simulink model "ULInjurySubject_Biphasic_1Hz_08102023"  (R2023a)
settings: Solver=VariableStepAuto  StartTime=0.0  StopTime=2000  RelTol=1e-3
values from neighbouring files (symbols this model uses):
  Cn = 1    [Inhibitory_excitatory_ULInjury_1Hz_08102023.m]    (also in Inhibitory_excitatory_ULInjury_30Hz_08102023.m; InitialExcitatoryInhibitoryNeurons_Healthy08062023.m; InitialExcitatoryInhibitoryULInjured_08102023_DSD.m)
  EKEx = -90    [Inhibitory_excitatory_ULInjury_1Hz_08102023.m]    (also in Inhibitory_excitatory_ULInjury_30Hz_08102023.m; InitialExcitatoryInhibitoryNeurons_Healthy08062023.m; InitialExcitatoryInhibitoryULInjured_08102023_DSD.m)
  EKIn = -90    [Inhibitory_excitatory_ULInjury_1Hz_08102023.m]    (also in Inhibitory_excitatory_ULInjury_30Hz_08102023.m; InitialExcitatoryInhibitoryNeurons_Healthy08062023.m; InitialExcitatoryInhibitoryULInjured_08102023_DSD.m)
  ELEx = -65    [Inhibitory_excitatory_ULInjury_1Hz_08102023.m]    (also in Inhibitory_excitatory_ULInjury_30Hz_08102023.m; InitialExcitatoryInhibitoryNeurons_Healthy08062023.m; InitialExcitatoryInhibitoryULInjured_08102023_DSD.m)
  ELIn = -65    [Inhibitory_excitatory_ULInjury_1Hz_08102023.m]    (also in Inhibitory_excitatory_ULInjury_30Hz_08102023.m; InitialExcitatoryInhibitoryNeurons_Healthy08062023.m; InitialExcitatoryInhibitoryULInjured_08102023_DSD.m)
  ENaEx = 60    [Inhibitory_excitatory_ULInjury_1Hz_08102023.m]    (also in Inhibitory_excitatory_ULInjury_30Hz_08102023.m; InitialExcitatoryInhibitoryNeurons_Healthy08062023.m; InitialExcitatoryInhibitoryULInjured_08102023_DSD.m)
  ENaIn = 55    [Inhibitory_excitatory_ULInjury_1Hz_08102023.m]    (also in Inhibitory_excitatory_ULInjury_30Hz_08102023.m; InitialExcitatoryInhibitoryNeurons_Healthy08062023.m; InitialExcitatoryInhibitoryULInjured_08102023_DSD.m)
  ErestE = -65    [Inhibitory_excitatory_ULInjury_1Hz_08102023.m]    (also in Inhibitory_excitatory_ULInjury_30Hz_08102023.m; InitialExcitatoryInhibitoryNeurons_Healthy08062023.m; InitialExcitatoryInhibitoryULInjured_08102023_DSD.m)
  ErestIn = -64    [Inhibitory_excitatory_ULInjury_1Hz_08102023.m]    (also in Inhibitory_excitatory_ULInjury_30Hz_08102023.m; InitialExcitatoryInhibitoryNeurons_Healthy08062023.m; InitialExcitatoryInhibitoryULInjured_08102023_DSD.m)
  ESynE = -10    [Inhibitory_excitatory_ULInjury_1Hz_08102023.m]    (also in Inhibitory_excitatory_ULInjury_30Hz_08102023.m; InitialExcitatoryInhibitoryNeurons_Healthy08062023.m; InitialExcitatoryInhibitoryULInjured_08102023_DSD.m)
  ESynE2 = -10    [Inhibitory_excitatory_ULInjury_1Hz_08102023.m]    (also in Inhibitory_excitatory_ULInjury_30Hz_08102023.m; InitialExcitatoryInhibitoryNeurons_Healthy08062023.m; InitialExcitatoryInhibitoryULInjured_08102023_DSD.m)
  ESynE3 = -10    [Inhibitory_excitatory_ULInjury_1Hz_08102023.m]    (also in Inhibitory_excitatory_ULInjury_30Hz_08102023.m; InitialExcitatoryInhibitoryNeurons_Healthy08062023.m; InitialExcitatoryInhibitoryULInjured_08102023_DSD.m)
  ESynE4 = -10    [Inhibitory_excitatory_ULInjury_1Hz_08102023.m]    (also in Inhibitory_excitatory_ULInjury_30Hz_08102023.m; InitialExcitatoryInhibitoryNeurons_Healthy08062023.m; InitialExcitatoryInhibitoryULInjured_08102023_DSD.m)
  ESynE5 = -10    [Inhibitory_excitatory_ULInjury_1Hz_08102023.m]    (also in Inhibitory_excitatory_ULInjury_30Hz_08102023.m; InitialExcitatoryInhibitoryNeurons_Healthy08062023.m; InitialExcitatoryInhibitoryULInjured_08102023_DSD.m)
  ESynE610 = -24    [Inhibitory_excitatory_ULInjury_1Hz_08102023.m]    (also in Inhibitory_excitatory_ULInjury_30Hz_08102023.m; InitialExcitatoryInhibitoryNeurons_Healthy08062023.m; InitialExcitatoryInhibitoryULInjured_08102023_DSD.m)
  ESynE6p = -10    [Inhibitory_excitatory_ULInjury_1Hz_08102023.m]    (also in Inhibitory_excitatory_ULInjury_30Hz_08102023.m; InitialExcitatoryInhibitoryNeurons_Healthy08062023.m; InitialExcitatoryInhibitoryULInjured_08102023_DSD.m)
  ESynI2 = -80    [Inhibitory_excitatory_ULInjury_1Hz_08102023.m]    (also in Inhibitory_excitatory_ULInjury_30Hz_08102023.m; InitialExcitatoryInhibitoryNeurons_Healthy08062023.m; InitialExcitatoryInhibitoryULInjured_08102023_DSD.m)
  ESynI3 = -80    [Inhibitory_excitatory_ULInjury_1Hz_08102023.m]    (also in Inhibitory_excitatory_ULInjury_30Hz_08102023.m; InitialExcitatoryInhibitoryNeurons_Healthy08062023.m; InitialExcitatoryInhibitoryULInjured_08102023_DSD.m)
  ESynI5 = -80    [Inhibitory_excitatory_ULInjury_1Hz_08102023.m]    (also in Inhibitory_excitatory_ULInjury_30Hz_08102023.m; InitialExcitatoryInhibitoryNeurons_Healthy08062023.m; InitialExcitatoryInhibitoryULInjured_08102023_DSD.m)
  ESynI6p = -82    [Inhibitory_excitatory_ULInjury_1Hz_08102023.m]    (also in Inhibitory_excitatory_ULInjury_30Hz_08102023.m; InitialExcitatoryInhibitoryNeurons_Healthy08062023.m; InitialExcitatoryInhibitoryULInjured_08102023_DSD.m)
  Exh0 = ahEx(V0)./(ahEx(V0)+bhEx(V0))    [Inhibitory_excitatory_ULInjury_1Hz_08102023.m]    (also in Inhibitory_excitatory_ULInjury_30Hz_08102023.m; InitialExcitatoryInhibitoryNeurons_Healthy08062023.m; InitialExcitatoryInhibitoryULInjured_08102023_DSD.m)
  Exm0 = amEx(V0)./(amEx(V0)+bmEx(V0))    [Inhibitory_excitatory_ULInjury_1Hz_08102023.m]    (also in Inhibitory_excitatory_ULInjury_30Hz_08102023.m; InitialExcitatoryInhibitoryNeurons_Healthy08062023.m; InitialExcitatoryInhibitoryULInjured_08102023_DSD.m)
  Exn0 = anEx(V0)./(anEx(V0)+bnEx(V0))    [Inhibitory_excitatory_ULInjury_1Hz_08102023.m]    (also in Inhibitory_excitatory_ULInjury_30Hz_08102023.m; InitialExcitatoryInhibitoryNeurons_Healthy08062023.m; InitialExcitatoryInhibitoryULInjured_08102023_DSD.m)
  gKEx = 100    [Inhibitory_excitatory_ULInjury_1Hz_08102023.m]    (also in Inhibitory_excitatory_ULInjury_30Hz_08102023.m; InitialExcitatoryInhibitoryNeurons_Healthy08062023.m; InitialExcitatoryInhibitoryULInjured_08102023_DSD.m)
  gKIn = 9    [Inhibitory_excitatory_ULInjury_1Hz_08102023.m]    (also in Inhibitory_excitatory_ULInjury_30Hz_08102023.m; InitialExcitatoryInhibitoryNeurons_Healthy08062023.m; InitialExcitatoryInhibitoryULInjured_08102023_DSD.m)
  gLEx = 0.1    [Inhibitory_excitatory_ULInjury_1Hz_08102023.m]    (also in Inhibitory_excitatory_ULInjury_30Hz_08102023.m; InitialExcitatoryInhibitoryNeurons_Healthy08062023.m; InitialExcitatoryInhibitoryULInjured_08102023_DSD.m)
  gLIn = 0.1    [Inhibitory_excitatory_ULInjury_1Hz_08102023.m]    (also in Inhibitory_excitatory_ULInjury_30Hz_08102023.m; InitialExcitatoryInhibitoryNeurons_Healthy08062023.m; InitialExcitatoryInhibitoryULInjured_08102023_DSD.m)
  gNaEx = 30    [Inhibitory_excitatory_ULInjury_1Hz_08102023.m]    (also in Inhibitory_excitatory_ULInjury_30Hz_08102023.m; InitialExcitatoryInhibitoryNeurons_Healthy08062023.m; InitialExcitatoryInhibitoryULInjured_08102023_DSD.m)
  gNaIn = 35    [Inhibitory_excitatory_ULInjury_1Hz_08102023.m]    (also in Inhibitory_excitatory_ULInjury_30Hz_08102023.m; InitialExcitatoryInhibitoryNeurons_Healthy08062023.m; InitialExcitatoryInhibitoryULInjured_08102023_DSD.m)
  gSynE = 0.08    [Inhibitory_excitatory_ULInjury_1Hz_08102023.m]    (also in Inhibitory_excitatory_ULInjury_30Hz_08102023.m; InitialExcitatoryInhibitoryNeurons_Healthy08062023.m; InitialExcitatoryInhibitoryULInjured_08102023_DSD.m)
  gSynE2 = 0.08    [Inhibitory_excitatory_ULInjury_1Hz_08102023.m]    (also in Inhibitory_excitatory_ULInjury_30Hz_08102023.m; InitialExcitatoryInhibitoryNeurons_Healthy08062023.m; InitialExcitatoryInhibitoryULInjured_08102023_DSD.m)
  gSynE3 = 0.08    [Inhibitory_excitatory_ULInjury_1Hz_08102023.m]    (also in Inhibitory_excitatory_ULInjury_30Hz_08102023.m; InitialExcitatoryInhibitoryNeurons_Healthy08062023.m; InitialExcitatoryInhibitoryULInjured_08102023_DSD.m)
  gSynE4 = 0.08    [Inhibitory_excitatory_ULInjury_1Hz_08102023.m]    (also in Inhibitory_excitatory_ULInjury_30Hz_08102023.m; InitialExcitatoryInhibitoryNeurons_Healthy08062023.m; InitialExcitatoryInhibitoryULInjured_08102023_DSD.m)
  gSynE5 = 0.08    [Inhibitory_excitatory_ULInjury_1Hz_08102023.m]    (also in Inhibitory_excitatory_ULInjury_30Hz_08102023.m; InitialExcitatoryInhibitoryNeurons_Healthy08062023.m; InitialExcitatoryInhibitoryULInjured_08102023_DSD.m)
  gSynE6 = 0.08    [Inhibitory_excitatory_ULInjury_1Hz_08102023.m]    (also in Inhibitory_excitatory_ULInjury_30Hz_08102023.m; InitialExcitatoryInhibitoryNeurons_Healthy08062023.m; InitialExcitatoryInhibitoryULInjured_08102023_DSD.m)
  gSynI2 = 0.12    [Inhibitory_excitatory_ULInjury_1Hz_08102023.m]    (also in Inhibitory_excitatory_ULInjury_30Hz_08102023.m; InitialExcitatoryInhibitoryNeurons_Healthy08062023.m; InitialExcitatoryInhibitoryULInjured_08102023_DSD.m)
  gSynI3 = 0.12    [Inhibitory_excitatory_ULInjury_1Hz_08102023.m]    (also in Inhibitory_excitatory_ULInjury_30Hz_08102023.m; InitialExcitatoryInhibitoryNeurons_Healthy08062023.m; InitialExcitatoryInhibitoryULInjured_08102023_DSD.m)
  gSynI5 = 0.12    [Inhibitory_excitatory_ULInjury_1Hz_08102023.m]    (also in Inhibitory_excitatory_ULInjury_30Hz_08102023.m; InitialExcitatoryInhibitoryNeurons_Healthy08062023.m; InitialExcitatoryInhibitoryULInjured_08102023_DSD.m)
  gSynI6 = 0.12    [Inhibitory_excitatory_ULInjury_1Hz_08102023.m]    (also in Inhibitory_excitatory_ULInjury_30Hz_08102023.m; InitialExcitatoryInhibitoryNeurons_Healthy08062023.m; InitialExcitatoryInhibitoryULInjured_08102023_DSD.m)
  Inh0 = ahIn(ErestIn)./(ahIn(ErestIn)+bhIn(ErestIn))    [Inhibitory_excitatory_ULInjury_1Hz_08102023.m]    (also in Inhibitory_excitatory_ULInjury_30Hz_08102023.m; InitialExcitatoryInhibitoryNeurons_Healthy08062023.m; InitialExcitatoryInhibitoryULInjured_08102023_DSD.m)
  Inm0 = amIn(ErestIn)./(amIn(ErestIn)+bmIn(ErestIn))    [Inhibitory_excitatory_ULInjury_1Hz_08102023.m]    (also in Inhibitory_excitatory_ULInjury_30Hz_08102023.m; InitialExcitatoryInhibitoryNeurons_Healthy08062023.m; InitialExcitatoryInhibitoryULInjured_08102023_DSD.m)
  Inn0 = anIn(ErestIn)./(anIn(ErestIn)+bnIn(ErestIn))    [Inhibitory_excitatory_ULInjury_1Hz_08102023.m]    (also in Inhibitory_excitatory_ULInjury_30Hz_08102023.m; InitialExcitatoryInhibitoryNeurons_Healthy08062023.m; InitialExcitatoryInhibitoryULInjured_08102023_DSD.m)
  TawIExt = 30    [Inhibitory_excitatory_ULInjury_1Hz_08102023.m]    (also in Inhibitory_excitatory_ULInjury_30Hz_08102023.m; InitialExcitatoryInhibitoryNeurons_Healthy08062023.m = 200; InitialExcitatoryInhibitoryULInjured_08102023_DSD.m = 200)
  TawIExtE = 30    [Inhibitory_excitatory_ULInjury_1Hz_08102023.m]    (also in Inhibitory_excitatory_ULInjury_30Hz_08102023.m; InitialExcitatoryInhibitoryNeurons_Healthy08062023.m = 1; InitialExcitatoryInhibitoryULInjured_08102023_DSD.m = 10)
  TawSynE = 5    [Inhibitory_excitatory_ULInjury_1Hz_08102023.m]    (also in Inhibitory_excitatory_ULInjury_30Hz_08102023.m; InitialExcitatoryInhibitoryNeurons_Healthy08062023.m; InitialExcitatoryInhibitoryULInjured_08102023_DSD.m)
  TawSynE10 = 5    [Inhibitory_excitatory_ULInjury_1Hz_08102023.m]    (also in Inhibitory_excitatory_ULInjury_30Hz_08102023.m; InitialExcitatoryInhibitoryNeurons_Healthy08062023.m; InitialExcitatoryInhibitoryULInjured_08102023_DSD.m = 3)
  TawSynE2 = 11    [Inhibitory_excitatory_ULInjury_1Hz_08102023.m]    (also in Inhibitory_excitatory_ULInjury_30Hz_08102023.m; InitialExcitatoryInhibitoryNeurons_Healthy08062023.m = 12; InitialExcitatoryInhibitoryULInjured_08102023_DSD.m = 5)
  TawSynE3 = 10    [Inhibitory_excitatory_ULInjury_1Hz_08102023.m]    (also in Inhibitory_excitatory_ULInjury_30Hz_08102023.m; InitialExcitatoryInhibitoryNeurons_Healthy08062023.m = 18; InitialExcitatoryInhibitoryULInjured_08102023_DSD.m = 8)
  TawSynE4 = 6    [Inhibitory_excitatory_ULInjury_1Hz_08102023.m]    (also in Inhibitory_excitatory_ULInjury_30Hz_08102023.m; InitialExcitatoryInhibitoryNeurons_Healthy08062023.m; InitialExcitatoryInhibitoryULInjured_08102023_DSD.m)
  TawSynE41 = 14    [Inhibitory_excitatory_ULInjury_1Hz_08102023.m]    (also in Inhibitory_excitatory_ULInjury_30Hz_08102023.m; InitialExcitatoryInhibitoryNeurons_Healthy08062023.m = 15; InitialExcitatoryInhibitoryULInjured_08102023_DSD.m = 6)
  TawSynE5 = 6    [Inhibitory_excitatory_ULInjury_1Hz_08102023.m]    (also in Inhibitory_excitatory_ULInjury_30Hz_08102023.m; InitialExcitatoryInhibitoryNeurons_Healthy08062023.m; InitialExcitatoryInhibitoryULInjured_08102023_DSD.m)
  TawSynE6 = 3    [Inhibitory_excitatory_ULInjury_1Hz_08102023.m]    (also in Inhibitory_excitatory_ULInjury_30Hz_08102023.m; InitialExcitatoryInhibitoryNeurons_Healthy08062023.m; InitialExcitatoryInhibitoryULInjured_08102023_DSD.m)
  TawSynE66E = 5    [Inhibitory_excitatory_ULInjury_1Hz_08102023.m]    (also in Inhibitory_excitatory_ULInjury_30Hz_08102023.m; InitialExcitatoryInhibitoryNeurons_Healthy08062023.m; InitialExcitatoryInhibitoryULInjured_08102023_DSD.m)
  TawSynI2 = 1    [Inhibitory_excitatory_ULInjury_1Hz_08102023.m]    (also in Inhibitory_excitatory_ULInjury_30Hz_08102023.m; InitialExcitatoryInhibitoryNeurons_Healthy08062023.m; InitialExcitatoryInhibitoryULInjured_08102023_DSD.m = 2)
  TawSynI3 = 30    [Inhibitory_excitatory_ULInjury_1Hz_08102023.m]    (also in Inhibitory_excitatory_ULInjury_30Hz_08102023.m; InitialExcitatoryInhibitoryNeurons_Healthy08062023.m = 35; InitialExcitatoryInhibitoryULInjured_08102023_DSD.m)
  TawSynI5 = 4    [Inhibitory_excitatory_ULInjury_1Hz_08102023.m]    (also in Inhibitory_excitatory_ULInjury_30Hz_08102023.m; InitialExcitatoryInhibitoryNeurons_Healthy08062023.m = 1; InitialExcitatoryInhibitoryULInjured_08102023_DSD.m = 1)
  TawSynI6 = 3    [Inhibitory_excitatory_ULInjury_1Hz_08102023.m]    (also in Inhibitory_excitatory_ULInjury_30Hz_08102023.m; InitialExcitatoryInhibitoryNeurons_Healthy08062023.m; InitialExcitatoryInhibitoryULInjured_08102023_DSD.m)
  V0 = -65    [Inhibitory_excitatory_ULInjury_1Hz_08102023.m]    (also in Inhibitory_excitatory_ULInjury_30Hz_08102023.m; InitialExcitatoryInhibitoryNeurons_Healthy08062023.m; InitialExcitatoryInhibitoryULInjured_08102023_DSD.m)
  V0In = -64    [Inhibitory_excitatory_ULInjury_1Hz_08102023.m]    (also in Inhibitory_excitatory_ULInjury_30Hz_08102023.m; InitialExcitatoryInhibitoryNeurons_Healthy08062023.m; InitialExcitatoryInhibitoryULInjured_08102023_DSD.m)
  w10 = 0.035    [Inhibitory_excitatory_ULInjury_1Hz_08102023.m]    (also in Inhibitory_excitatory_ULInjury_30Hz_08102023.m; InitialExcitatoryInhibitoryNeurons_Healthy08062023.m)
  w12 = -0.2    [Inhibitory_excitatory_ULInjury_1Hz_08102023.m]    (also in Inhibitory_excitatory_ULInjury_30Hz_08102023.m; InitialExcitatoryInhibitoryNeurons_Healthy08062023.m = -0.28; InitialExcitatoryInhibitoryULInjured_08102023_DSD.m = -0.35)
  w14 = 0.05    [Inhibitory_excitatory_ULInjury_1Hz_08102023.m]    (also in Inhibitory_excitatory_ULInjury_30Hz_08102023.m; InitialExcitatoryInhibitoryNeurons_Healthy08062023.m = 0.09; InitialExcitatoryInhibitoryULInjured_08102023_DSD.m = 0.09)
  w15 = -0.45    [Inhibitory_excitatory_ULInjury_1Hz_08102023.m]    (also in Inhibitory_excitatory_ULInjury_30Hz_08102023.m = -0.07; InitialExcitatoryInhibitoryNeurons_Healthy08062023.m = -0.4; InitialExcitatoryInhibitoryULInjured_08102023_DSD.m = -0.4)
  w26 = 0.2    [Inhibitory_excitatory_ULInjury_1Hz_08102023.m]    (also in Inhibitory_excitatory_ULInjury_30Hz_08102023.m = 0.25; InitialExcitatoryInhibitoryNeurons_Healthy08062023.m = 0.05; InitialExcitatoryInhibitoryULInjured_08102023_DSD.m = 0.05)
  w28 = 0.165    [Inhibitory_excitatory_ULInjury_1Hz_08102023.m]    (also in Inhibitory_excitatory_ULInjury_30Hz_08102023.m; InitialExcitatoryInhibitoryNeurons_Healthy08062023.m = 0.13; InitialExcitatoryInhibitoryULInjured_08102023_DSD.m = 0.13)
  w34 = 0.09    [Inhibitory_excitatory_ULInjury_1Hz_08102023.m]    (also in Inhibitory_excitatory_ULInjury_30Hz_08102023.m; InitialExcitatoryInhibitoryNeurons_Healthy08062023.m = 0.03; InitialExcitatoryInhibitoryULInjured_08102023_DSD.m = 0.06)
  w63 = -0.12    [Inhibitory_excitatory_ULInjury_1Hz_08102023.m]    (also in Inhibitory_excitatory_ULInjury_30Hz_08102023.m; InitialExcitatoryInhibitoryNeurons_Healthy08062023.m = -0.08; InitialExcitatoryInhibitoryULInjured_08102023_DSD.m = -0.27)
  w66E = 0.2    [Inhibitory_excitatory_ULInjury_1Hz_08102023.m]    (also in Inhibitory_excitatory_ULInjury_30Hz_08102023.m; InitialExcitatoryInhibitoryNeurons_Healthy08062023.m = 0.09; InitialExcitatoryInhibitoryULInjured_08102023_DSD.m = 0.1)
  w67 = -0.4    [Inhibitory_excitatory_ULInjury_1Hz_08102023.m]    (also in Inhibitory_excitatory_ULInjury_30Hz_08102023.m; InitialExcitatoryInhibitoryNeurons_Healthy08062023.m = -0.55; InitialExcitatoryInhibitoryULInjured_08102023_DSD.m = -0.55)
  w68 = 0.35    [Inhibitory_excitatory_ULInjury_1Hz_08102023.m]    (also in Inhibitory_excitatory_ULInjury_30Hz_08102023.m; InitialExcitatoryInhibitoryNeurons_Healthy08062023.m = 0.1; InitialExcitatoryInhibitoryULInjured_08102023_DSD.m = 0.1)
  w71 = 0.25    [Inhibitory_excitatory_ULInjury_1Hz_08102023.m]    (also in Inhibitory_excitatory_ULInjury_30Hz_08102023.m; InitialExcitatoryInhibitoryNeurons_Healthy08062023.m; InitialExcitatoryInhibitoryULInjured_08102023_DSD.m)
  w83 = 0.2    [Inhibitory_excitatory_ULInjury_1Hz_08102023.m]    (also in Inhibitory_excitatory_ULInjury_30Hz_08102023.m; InitialExcitatoryInhibitoryNeurons_Healthy08062023.m = 0.13; InitialExcitatoryInhibitoryULInjured_08102023_DSD.m = 0.08)
  w85 = 0.1    [Inhibitory_excitatory_ULInjury_1Hz_08102023.m]    (also in Inhibitory_excitatory_ULInjury_30Hz_08102023.m = 0.12; InitialExcitatoryInhibitoryNeurons_Healthy08062023.m = 0.04; InitialExcitatoryInhibitoryULInjured_08102023_DSD.m = 0.05)
(part 1 of 5)
settings Model: Creator=mfard  LastModifiedBy=mfard
settings SolverCC: AlgebraicLoopSolver=TrustRegion
settings DebuggingCC: UnconnectedInputMsg=warning  UnconnectedOutputMsg=warning  UnconnectedLineMsg=warning
settings ModelReferenceCC: EnableRefExpFcnMdlSchedulingChecks=on

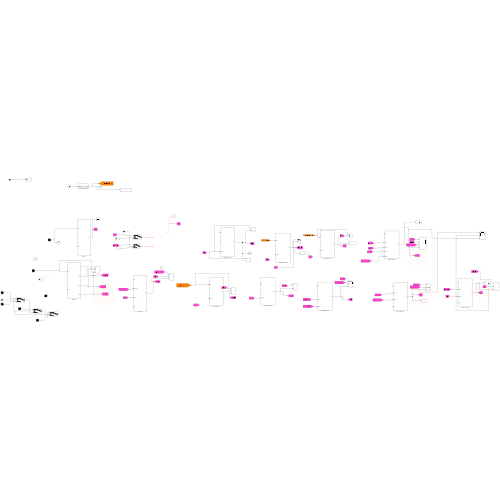
[thumbnail: Simulink's stored preview of the top-level diagram]
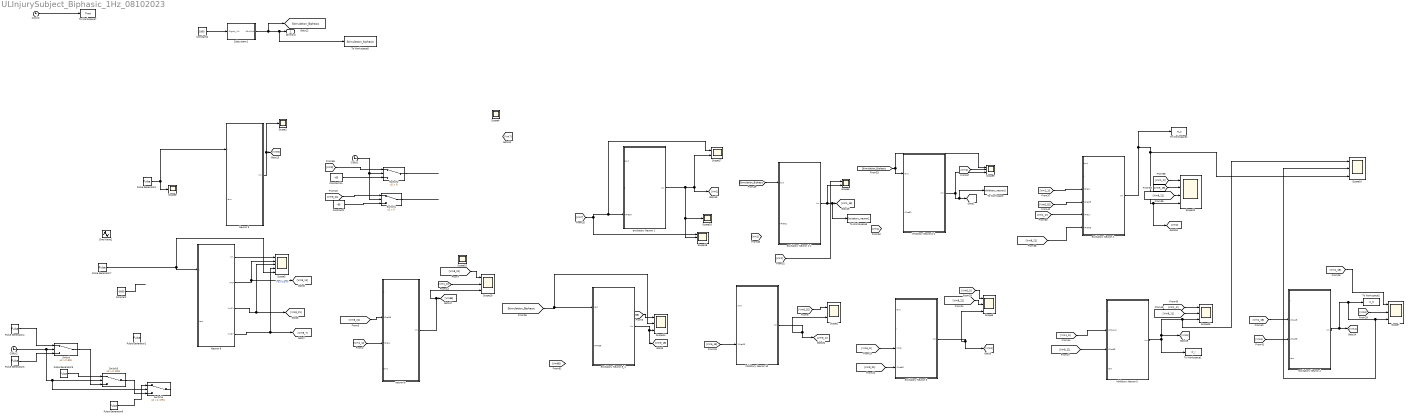
== system ULInjurySubject_Biphasic_1Hz_08102023 ==
  Clock1 : Clock
  Clock2 : Clock
  Clock3 : Clock
  Constant : Constant  Value=-5000
  Constant1 : Constant  Value=-65
  Constant14 : Constant  Value=-65
  Constant2 : Constant  Value=1000
  Inhibitory Neuron 10 : Subsystem
      mask init:
      | p=1
  Inhibitory Neuron 5 : Subsystem
      mask init:
      | p=1
  Inhibitory Neuron1-1 : Subsystem
      mask init:
      | p=1
  Neuron 6 : Subsystem
      mask init:
      | p=1
  Neuron 8 : Subsystem
      mask init:
      | p=1
  Neuron 9 : Subsystem
      mask init:
      | p=1
  Pulse Generator1 : DiscretePulseGenerator  PulseType=Time based  Amplitude=170  Period=15  PulseWidth=2
  Pulse Generator2 : DiscretePulseGenerator  PulseType=Time based  Amplitude=20  Period=20  PulseWidth=5
  Pulse Generator3 : DiscretePulseGenerator  PulseType=Time based  Amplitude=100  Period=150
  Pulse Generator4 : DiscretePulseGenerator  PulseType=Time based  Amplitude=175  Period=100
  Pulse Generator5 : DiscretePulseGenerator  PulseType=Time based  Amplitude=200  Period=40
  Pulse Generator6 : DiscretePulseGenerator  PulseType=Time based  Amplitude=250  Period=24
  Pulse Generator7 : DiscretePulseGenerator  PulseType=Time based  Amplitude=200  Period=22
  Scope{1,4,8,15..16} (5 alike) : Scope
  Scope{5,7,9..10,14,18..19,25} (8 alike) : Scope  NumInputPorts=3
  Scope12 : Scope  NumInputPorts=4
  Scope17 : Scope  NumInputPorts=2
  Scope2 : Scope  NumInputPorts=2
  Scope3 : Scope  NumInputPorts=5
  Scope6 : Scope  NumInputPorts=2
  Sine Wave2 : Sin  Amplitude=5  Frequency=0.1*pi  SampleTime=0
  Subsystem1 : Subsystem
  Switch : Switch  Threshold=601  SaturateOnIntegerOverflow=off  InputSameDT=off
  Switch1 : Switch  Criteria=u2 > Threshold  SaturateOnIntegerOverflow=off  InputSameDT=off
  Switch2 : Switch  Criteria=u2 > Threshold  SaturateOnIntegerOverflow=off  InputSameDT=off
  Switch3 : Switch  Threshold=1001  SaturateOnIntegerOverflow=off  InputSameDT=off
  Switch4 : Switch  Threshold=1751  SaturateOnIntegerOverflow=off  InputSameDT=off
  To Workspace : ToWorkspace  VariableName=Inhibitory_neuron1  SaveFormat=Timeseries  SampleTime=-1
  To Workspace1 : ToWorkspace  VariableName=w_i  SampleTime=-1
  To Workspace2 : ToWorkspace  VariableName=w_e  SampleTime=-1
  To Workspace3 : ToWorkspace  VariableName=Excitatory_neuron1  SaveFormat=Timeseries  SampleTime=-1
  To Workspace4 : ToWorkspace  VariableName=w_s  SampleTime=-1
  To Workspace5 : ToWorkspace  VariableName=Stimulation_biphasic  SampleTime=-1
  To Workspace7 : ToWorkspace  VariableName=Time  SampleTime=-1
  excitatory Neuron 1 : Subsystem
      mask init:
      | p=1
  excitatory Neuron 1-1 : Subsystem
      mask init:
      | p=1
  excitatory Neuron 2 : Subsystem
      mask init:
      | p=1
  excitatory Neuron 3 : Subsystem
      mask init:
      | p=1
  excitatory Neuron 4 : Subsystem
      mask init:
      | p=1
  excitatory Neuron 6_1 : Subsystem
      mask init:
      | p=1
  StimOut : Outport
  tag scope: Stimulation_Biphasic=global
  wires:
  Neuron 6/1(Vm) -> Scope19/3, [Vm6E]
  [Vm8_21] -> Scope19/1
  [Vm6_1E] -> Scope2/1
  excitatory Neuron 6_1/1(Vm) -> [Vm6_1E], Scope14/3
  [Vm1] -> Scope6/1
  Pulse Generator3/1 -> Switch/3
  Pulse Generator6/1 -> Switch4/1
  Switch3/1 -> Switch4/3
  [Vm6E] -> Scope14/1
  [Vm1_1I] -> Scope19/2
  Clock2/1 -> Switch4/2, Switch3/2, Switch/2
  Switch/1 -> Switch3/3
  Inhibitory Neuron 10/1(Vm) -> Scope2/2, [Vm6_1I]
  Inhibitory Neuron1-1/1(Vm) -> Scope9/3, To Workspace/1, [Vm1_1I]
  [Vm8_21] -> Neuron 6/2(VPre8E)
  Clock3/1 -> To Workspace7/1
  [Vm6_1E] -> Inhibitory Neuron 10/2(VPre6E)
  Pulse Generator5/1 -> Switch3/1
  [Vm1] -> Scope9/2
  Pulse Generator4/1 -> Switch/1
  [Vm1_1I] -> Neuron 6/3(VPre1I)
  excitatory Neuron 1-1/1(Vm) -> Scope6/2, To Workspace3/1, [Vm1_1E]
  Subsystem1/1(StimOut) -> [Stimulation_Biphasic], To Workspace5/1, StimOut/1
  Constant2/1 -> Subsystem1/1(Signal_in1)
  Neuron 8/2(Vm5) -> [Vm8_11], Scope3/2  "Input Signal"
  Neuron 8/3(Vm21) -> Scope3/3, [Vm8_21]
  Neuron 8/4(Vm87) -> Scope3/4, [Vm8_7]
  Neuron 8/1(Vm) -> Scope3/1
  Pulse Generator7/1 -> Neuron 8/1("I "), Scope3/5
  Constant/1 -> ?
  Constant1/1 -> Switch1/3
  ? -> Scope4/1, [Vm7]
  Pulse Generator1/1 -> Scope8/1, Neuron 9/1("I ")
  Neuron 9/1(Vm) -> Scope1/1, [Vm9]
  Constant14/1 -> Switch2/3
  Switch1/1 -> ?
  Clock1/1 -> Switch1/2, Switch2/2
  Switch2/1 -> ?
  [Vm8_21] -> Switch1/1
  [Vm9] -> Switch2/1
  excitatory Neuron 1/1(Vm) -> Scope17/2, [Vm1], Scope16/1, Scope18/2
  [Vm7] -> Scope17/1, excitatory Neuron 1/3(VPreE7), Scope18/1
  [Vm6_1E] -> excitatory Neuron 2/4(VPre6E)
  [Vm8_21] -> Scope12/3
  [Vm1_1I] -> excitatory Neuron 2/3("VPre1I ")
  [Vm8_21] -> excitatory Neuron 2/6(VPre8E)
  excitatory Neuron 2/1(Vm) -> To Workspace4/1, Scope10/3, [Vm2], Scope12/4
  [Vm1_1I] -> excitatory Neuron 2/5(VPre1I)
  [Vm1_1I] -> Scope12/1
  [Vm6_1E] -> Scope12/2
  [Vm8_21] -> excitatory Neuron 3/4(VPre8E)
  excitatory Neuron 3/1(Vm) -> Scope5/3, [Vm3]
  [Vm6_1I] -> Scope5/1
  [Vm6_1I] -> excitatory Neuron 3/3("VPreI ")
  [Vm8_21] -> Scope5/2
  [Vm8_11] -> Inhibitory Neuron 5/3(VPre8E)
  [Vm1_1I] -> Scope25/1
  [Vm3] -> Scope7/2
  [Vm1_1I] -> Inhibitory Neuron 5/2("VPre1_1I ")
  excitatory Neuron 4/1(Vm) -> Scope10/2, Scope7/3, To Workspace2/1, [Vm4]
  [Vm3] -> excitatory Neuron 4/3(VPre3E)
  Inhibitory Neuron 5/1(Vm) -> Scope10/1, Scope25/3, [Vm5], To Workspace1/1
  [Vm1_1E] -> Scope7/1
  [Vm1_1E] -> excitatory Neuron 4/2("VPre1E ")
  [Vm8_11] -> Scope25/2
  [Stimulation_Biphasic] -> Scope9/1, Inhibitory Neuron1-1/1(Iext)
  [Stimulation_Biphasic] -> excitatory Neuron 6_1/1(Iext), Scope14/2
  [Stimulation_Biphasic] -> excitatory Neuron 1-1/1(Iext)

== system ULInjurySubject_Biphasic_1Hz_08102023/Inhibitory Neuron 10 ==
  Iext : Inport
  VPre6E : Inport  Port=2
  Add : Sum  Inputs=+---+--
  Add1 : Sum  Inputs=+-
  Constant2 : Constant  Value=ENaIn
  Divide : Product  Inputs=**
  Gain : Gain  Gain=1/Cn
  Integrator : Integrator  InitialCondition=-64
  Ks : Subsystem
  Lk : Subsystem
  Naf : Subsystem
  Nap2 : Subsystem
  Scope{1..6} (6 alike) : Scope
  Subsystem : Subsystem
  Transfer Fcn1 : TransferFcn  Denominator=[TawIExt 1]
  Vm : Outport  VectorParamsAs1DForOutWhenUnconnected=off
  wires:
  Divide/1 -> Add/1
  Naf/1("INaf ") -> Scope4/1, Add/2
  Add/1 -> Scope3/1, Gain/1
  Transfer Fcn1/1 -> Scope1/1, Divide/2
  Gain/1 -> Integrator/1
  Subsystem/1(ku) -> Transfer Fcn1/1
  Iext/1 -> Subsystem/1(Iext)
  Add1/1 -> Divide/1
  Constant2/1 -> Add1/1
  Nap2/1("ISynE ") -> Scope2/1, Add/6
  VPre6E/1 -> Nap2/2(Pre)
  Integrator/1 -> Add1/2, Naf/1(Vm), Ks/1(Vm), Lk/1(Vm), Nap2/1(V), Vm/1
  Lk/1(ILk) -> Scope5/1, Add/4
  Ks/1(IKs) -> Scope6/1, Add/3

== system ULInjurySubject_Biphasic_1Hz_08102023/Inhibitory Neuron 5 ==
  "I " : Inport
  "VPre1_1I " : Inport  Port=2
  VPre8E : Inport  Port=3
  Iext : Inport  Port=4
  Add : Sum  Inputs=+---+---
  Add1 : Sum  Inputs=+-
  Constant2 : Constant  Value=ENaEx
  Divide : Product  Inputs=**
  Gain : Gain  Gain=1/Cn
  Integrator : Integrator  InitialCondition=V0In
  Ks : Subsystem
  Lk : Subsystem
  Naf : Subsystem
  Nap1 : Subsystem
  Nap2 : Subsystem
  Nap3 : Subsystem
  Scope{1..3,5} (4 alike) : Scope
  Subsystem : Subsystem
  Transfer Fcn1 : TransferFcn  Denominator=[TawIExt 1]
  Vm : Outport  VectorParamsAs1DForOutWhenUnconnected=off
  wires:
  Divide/1 -> Add/1
  Ks/1(IKs) -> Add/3
  Naf/1("INaf ") -> Add/2
  Add/1 -> Scope3/1, Gain/1
  Gain/1 -> Integrator/1
  "I "/1 -> Add/5
  Lk/1(ILk) -> Scope5/1, Add/4
  "VPre1_1I "/1 -> Nap1/2(Pre), Nap2/2(Pre)
  VPre8E/1 -> Nap3/2(Pre)
  Nap2/1("ISynI ") -> Add/7
  Nap3/1("ISynE ") -> Add/8
  Subsystem/1(ku) -> Transfer Fcn1/1
  Integrator/1 -> Nap2/1(V), Vm/1, Nap3/1(V), Nap1/1(V), Add1/2, Naf/1(Vm), Ks/1(Vm), Lk/1(Vm)
  Add1/1 -> Divide/1
  Constant2/1 -> Add1/1
  Transfer Fcn1/1 -> Divide/2, Scope1/1
  Iext/1 -> Subsystem/1(Iext)

== system ULInjurySubject_Biphasic_1Hz_08102023/Inhibitory Neuron1-1 ==
  Iext : Inport
  VPreE1 : Inport  Port=2
  Add : Sum  Inputs=+----
  Add1 : Sum  Inputs=+-
  Constant2 : Constant  Value=ENaIn
  Divide : Product  Inputs=**
  Gain : Gain  Gain=1/Cn
  Integrator : Integrator  InitialCondition=-64.00  AbsoluteTolerance=1e-6
  Ks : Subsystem
  Lk : Subsystem
  Naf : Subsystem
  Nap1 : Subsystem
  Scope{1..7} (7 alike) : Scope
  Subsystem : Subsystem
  Transfer Fcn1 : TransferFcn  Denominator=[TawIExt 1]
  Vm : Outport  VectorParamsAs1DForOutWhenUnconnected=off
  wires:
  Divide/1 -> Add/1
  Naf/1("INaf ") -> Scope6/1, Add/2
  Add/1 -> Scope3/1, Gain/1
  Transfer Fcn1/1 -> Scope1/1, Divide/2
  Gain/1 -> Integrator/1
  Subsystem/1(ku) -> Transfer Fcn1/1
  Iext/1 -> Subsystem/1(Iext)
  Add1/1 -> Divide/1
  Constant2/1 -> Add1/1
  Integrator/1 -> Add1/2, Naf/1(Vm), Ks/1(Vm), Lk/1(Vm), Nap1/1(V), Vm/1, Scope2/1
  VPreE1/1 -> Nap1/2(Pre)
  Nap1/1("ISynE ") -> Scope7/1, Add/5
  Lk/1(ILk) -> Scope4/1, Add/4
  Ks/1(IKs) -> Scope5/1, Add/3

== system ULInjurySubject_Biphasic_1Hz_08102023/Neuron 6 ==
  "I " : Inport
  VPre8E : Inport  Port=2
  VPre1I : Inport  Port=3
  Iext : Inport  Port=4
  Add : Sum  Inputs=+---++---
  Add1 : Sum  Inputs=+-
  Constant2 : Constant  Value=ENaEx
  Divide : Product  Inputs=**
  Gain : Gain  Gain=1/Cn
  Integrator : Integrator  InitialCondition=-65
  Ks : Subsystem
  Lk : Subsystem
  Naf : Subsystem
  Nap1 : Subsystem
  Nap2 : Subsystem
  Scope{,1..5} (6 alike) : Scope
  Subsystem : Subsystem
  Transfer Fcn1 : TransferFcn  Denominator="[TawIExtE  1]"
  Vm : Outport  VectorParamsAs1DForOutWhenUnconnected=off
  wires:
  Divide/1 -> Scope/1, Add/1
  Ks/1(IKs) -> Add/3
  Naf/1("INaf ") -> Add/2
  Add/1 -> Scope3/1, Gain/1
  Gain/1 -> Integrator/1
  "I "/1 -> Add/5
  Nap2/1("ISynI ") -> Add/9, Scope2/1
  Nap1/1("ISynE ") -> Scope1/1, Add/8
  VPre1I/1 -> Nap2/2(Pre)
  VPre8E/1 -> Nap1/2(Pre)
  Lk/1(ILk) -> Add/4
  Add1/1 -> Divide/1
  Iext/1 -> Subsystem/1(Iext)
  Constant2/1 -> Add1/1
  Subsystem/1(ku) -> Scope5/1, Transfer Fcn1/1
  Transfer Fcn1/1 -> Divide/2, Scope4/1
  Integrator/1 -> Vm/1, Lk/1(Vm), Ks/1(Vm), Add1/2, Naf/1(Vm), Nap1/1(V), Nap2/1(V)

== system ULInjurySubject_Biphasic_1Hz_08102023/Neuron 8 ==
  "I " : Inport
  Iext : Inport  Port=2
  Add : Sum  Inputs=+---+
  Add1 : Sum  Inputs=+-
  Constant1 : Constant  Value=0.1
  Constant2 : Constant  Value=ENaEx
  Constant3 : Constant  Value=0.3
  Constant4 : Constant  Value=0.5
  Divide : Product  Inputs=**
  Gain : Gain  Gain=1/Cn
  Integrator : Integrator  InitialCondition=-65
  Ks : Subsystem
  Lk : Subsystem
  Naf : Subsystem
  Scope{,1..5} (6 alike) : Scope
  Subsystem : Subsystem
  Transfer Fcn1 : TransferFcn  Denominator="[TawIExtE  1]"
  Variable Time Delay : VariableTransportDelay  MaximumDelay=10000  InitialOutput=-65
  Variable Time Delay1 : VariableTransportDelay  MaximumDelay=10000  InitialOutput=-65
  Variable Time Delay2 : VariableTransportDelay  MaximumDelay=10000  InitialOutput=-65
  Vm : Outport  VectorParamsAs1DForOutWhenUnconnected=off
  Vm5 : Outport  Port=2  VectorParamsAs1DForOutWhenUnconnected=off
  Vm21 : Outport  Port=3  VectorParamsAs1DForOutWhenUnconnected=off
  Vm87 : Outport  Port=4  VectorParamsAs1DForOutWhenUnconnected=off
  wires:
  Divide/1 -> Scope/1, Add/1
  Ks/1(IKs) -> Add/3
  Naf/1("INaf ") -> Add/2
  Add/1 -> Scope3/1, Gain/1
  Gain/1 -> Integrator/1
  Integrator/1 -> Scope2/1, Vm/1, Naf/1(Vm), Ks/1(Vm), Lk/1(Vm), Variable Time Delay2/1, Variable Time Delay1/1, Variable Time Delay/1
  Lk/1(ILk) -> Add/4
  "I "/1 -> Add1/2, Add/5
  Constant2/1 -> Add1/1
  Iext/1 -> Subsystem/1(Iext)
  Subsystem/1(ku) -> Scope5/1, Transfer Fcn1/1
  Transfer Fcn1/1 -> Divide/2, Scope4/1
  Add1/1 -> Divide/1
  Variable Time Delay/1 -> Vm87/1
  Constant1/1 -> Variable Time Delay/2
  Variable Time Delay1/1 -> Vm5/1
  Constant3/1 -> Variable Time Delay1/2
  Variable Time Delay2/1 -> Vm21/1
  Constant4/1 -> Variable Time Delay2/2

== system ULInjurySubject_Biphasic_1Hz_08102023/Neuron 9 ==
  "I " : Inport
  Iext : Inport  Port=2
  Add : Sum  Inputs=+---+
  Add1 : Sum  Inputs=+-
  Constant2 : Constant  Value=ENaEx
  Divide : Product  Inputs=**
  Gain : Gain  Gain=1/Cn
  Integrator : Integrator  InitialCondition=-65  AbsoluteTolerance=1e-6
  Ks : Subsystem
  Lk : Subsystem
  Naf : Subsystem
  Scope : Scope
  Scope3 : Scope
  Scope4 : Scope
  Subsystem : Subsystem
  Transfer Fcn1 : TransferFcn  Denominator=[TawIExt 1]
  Vm : Outport  VectorParamsAs1DForOutWhenUnconnected=off
  wires:
  Divide/1 -> Add/1, Scope/1
  Ks/1(IKs) -> Add/3
  Naf/1("INaf ") -> Add/2
  Add/1 -> Scope3/1, Gain/1
  Gain/1 -> Integrator/1
  "I "/1 -> Add/5
  Lk/1(ILk) -> Add/4
  Constant2/1 -> Add1/1
  Transfer Fcn1/1 -> Divide/2, Scope4/1
  Add1/1 -> Divide/1
  Subsystem/1(ku) -> Transfer Fcn1/1
  Integrator/1 -> Vm/1, Lk/1(Vm), Ks/1(Vm), Add1/2, Naf/1(Vm)
  Iext/1 -> Subsystem/1(Iext)

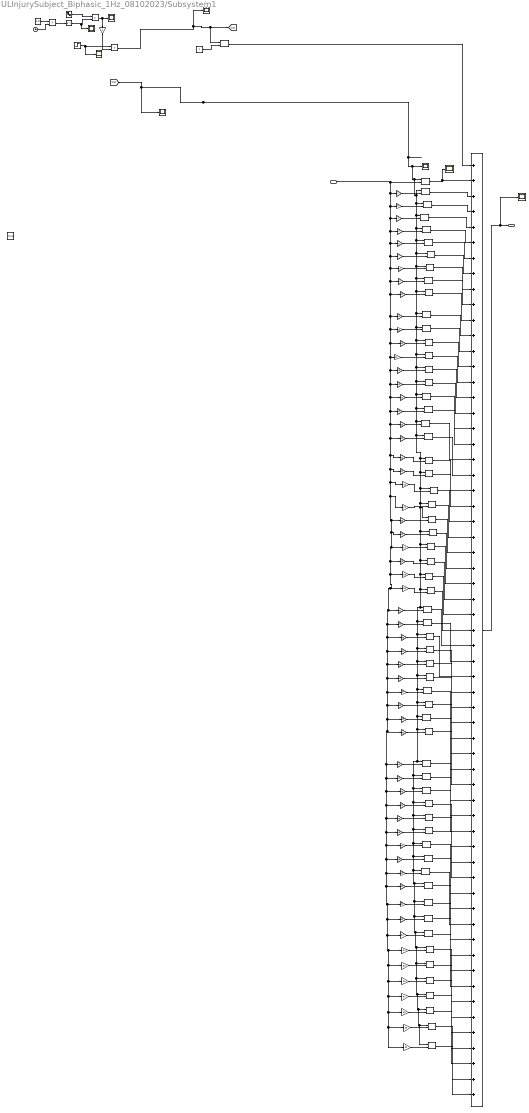
== system ULInjurySubject_Biphasic_1Hz_08102023/Subsystem1 ==
  Signal_in1 : Inport
  Add : Sum  Inputs=+++++++++++++++++++++++++++++++++++++++++++++++++++++++++++++
  Clock1 : Clock
  Constant1 : Constant  Value=-0.01
  Constant2 : Constant
  Divide3 : Product  Inputs=**
  Divide4 : Product  Inputs=**
  Divide5 : Product  Inputs=**
  Gain : Gain  Gain=2
  Gain1 : Gain  Gain=3
  Gain10 : Gain
  Gain12 : Gain  Gain=12
  Gain13 : Gain  Gain=13
  Gain14 : Gain  Gain=14
  Gain15 : Gain  Gain=15
  Gain16 : Gain  Gain=16
  Gain17 : Gain  Gain=17
  Gain18 : Gain  Gain=18
  Gain19 : Gain  Gain=19
  Gain2 : Gain  Gain=51
  Gain20 : Gain  Gain=20
  Gain21 : Gain  Gain=22
  Gain22 : Gain  Gain=23
  Gain23 : Gain  Gain=24
  Gain24 : Gain  Gain=25
  Gain25 : Gain  Gain=26
  Gain26 : Gain  Gain=27
  Gain27 : Gain  Gain=28
  Gain28 : Gain  Gain=29
  Gain29 : Gain  Gain=30
  Gain3 : Gain  Gain=52
  Gain30 : Gain  Gain=21
  Gain31 : Gain  Gain=32
  Gain32 : Gain  Gain=33
  Gain33 : Gain  Gain=34
  Gain34 : Gain  Gain=35
  Gain35 : Gain  Gain=36
  Gain36 : Gain  Gain=37
  Gain37 : Gain  Gain=38
  Gain38 : Gain  Gain=39
  Gain39 : Gain  Gain=40
  Gain4 : Gain  Gain=4
  Gain40 : Gain  Gain=31
  Gain41 : Gain  Gain=42
  Gain42 : Gain  Gain=43
  Gain43 : Gain  Gain=44
  Gain44 : Gain  Gain=45
  Gain45 : Gain  Gain=46
  Gain46 : Gain  Gain=47
  Gain47 : Gain  Gain=48
  Gain48 : Gain  Gain=49
  Gain49 : Gain  Gain=50
  Gain5 : Gain  Gain=5
  Gain50 : Gain  Gain=41
  Gain51 : Gain  Gain=53
  Gain52 : Gain  Gain=54
  Gain53 : Gain  Gain=55
  Gain54 : Gain  Gain=56
  Gain55 : Gain  Gain=57
  Gain56 : Gain  Gain=58
  Gain57 : Gain  Gain=59
  Gain58 : Gain  Gain=60
  Gain59 : Gain  Gain=10
  Gain6 : Gain  Gain=6
  Gain60 : Gain  Gain=11
  Gain7 : Gain  Gain=7
  Gain8 : Gain  Gain=8
  Gain9 : Gain  Gain=9
  Math Function1 : Math  SignedPower=on
  Pulse Generator : DiscretePulseGenerator  PulseType=Time based  Amplitude=100  Period=1000  PulseWidth=0.021
  Scope{1..7,24} (8 alike) : Scope
  Sine Wave2 : Sin  Amplitude=10500  Frequency=7.1*2*pi*2/3  Phase=pi/2  SampleTime=0
  Step1 : Step  Time=0.2112  Before=1  After=0  SampleTime=0
  Variable Time Delay{,1,3..9,19,29,39,49..60,81} (25 alike) : VariableTransportDelay  MaximumDelay=10000
  Variable Time Delay{2,11..18,20..28,30..38,40..48} (36 alike) : VariableTransportDelay  MaximumDelay=100000
  StimOut : Outport
  wires:
  Gain3/1 -> Variable Time Delay52/2
  Gain8/1 -> Variable Time Delay8/2
  Variable Time Delay1/1 -> Add/3
  Gain6/1 -> Variable Time Delay6/2
  Variable Time Delay46/1 -> Add/48
  Gain32/1 -> Variable Time Delay32/2
  Variable Time Delay54/1 -> Add/55
  Gain7/1 -> Variable Time Delay7/2
  Variable Time Delay34/1 -> Add/36
  Gain33/1 -> Variable Time Delay33/2
  Gain1/1 -> Variable Time Delay3/2
  Add/1 -> Scope2/1, StimOut/1
  Gain31/1 -> Variable Time Delay31/2
  Variable Time Delay6/1 -> Add/7
  Gain5/1 -> Variable Time Delay5/2
  Variable Time Delay47/1 -> Add/49
  Gain26/1 -> Variable Time Delay26/2
  Gain15/1 -> Variable Time Delay14/2
  Gain24/1 -> Variable Time Delay24/2
  Variable Time Delay24/1 -> Add/26
  Variable Time Delay12/1 -> Add/14
  Gain19/1 -> Variable Time Delay18/2
  Gain9/1 -> Variable Time Delay9/2
  Gain36/1 -> Variable Time Delay36/2
  Variable Time Delay15/1 -> Add/17
  Variable Time Delay50/1 -> Add/11
  Variable Time Delay36/1 -> Add/38
  Variable Time Delay37/1 -> Add/39
  Gain12/1 -> Variable Time Delay11/2
  Variable Time Delay22/1 -> Add/24
  Gain45/1 -> Variable Time Delay45/2
  Variable Time Delay4/1 -> Add/5
  Gain34/1 -> Variable Time Delay34/2
  Gain13/1 -> Variable Time Delay12/2
  Variable Time Delay44/1 -> Add/46
  Gain44/1 -> Variable Time Delay44/2
  Gain46/1 -> Variable Time Delay46/2
  Variable Time Delay13/1 -> Add/15
  Variable Time Delay33/1 -> Add/35
  Variable Time Delay14/1 -> Add/16
  Variable Time Delay45/1 -> Add/47
  Gain60/1 -> Variable Time Delay2/2
  Variable Time Delay29/1 -> Add/31
  Variable Time Delay7/1 -> Add/8
  Variable Time Delay8/1 -> Add/9
  Variable Time Delay48/1 -> Add/50
  Variable Time Delay39/1 -> Add/41
  Gain27/1 -> Variable Time Delay27/2
  Variable Time Delay32/1 -> Add/34
  Gain42/1 -> Variable Time Delay42/2
  Variable Time Delay31/1 -> Add/33
  Gain37/1 -> Variable Time Delay37/2
  Variable Time Delay5/1 -> Add/6
  Variable Time Delay18/1 -> Add/20
  Gain53/1 -> Variable Time Delay55/2
  Variable Time Delay57/1 -> Add/58
  Gain20/1 -> Variable Time Delay19/2
  Gain57/1 -> Variable Time Delay59/2
  Gain40/1 -> Variable Time Delay30/2
  Variable Time Delay20/1 -> Add/22
  Variable Time Delay55/1 -> Add/56
  Variable Time Delay2/1 -> Add/12
  Variable Time Delay58/1 -> Add/59
  Gain/1 -> Variable Time Delay1/2
  Variable Time Delay56/1 -> Add/57
  Gain16/1 -> Variable Time Delay15/2
  Variable Time Delay53/1 -> Add/54
  Variable Time Delay3/1 -> Add/4
  Gain52/1 -> Variable Time Delay54/2
  Variable Time Delay17/1 -> Add/19
  Variable Time Delay19/1 -> Add/21
  Gain56/1 -> Variable Time Delay58/2
  Gain2/1 -> Variable Time Delay51/2
  Gain48/1 -> Variable Time Delay48/2
  Variable Time Delay35/1 -> Add/37
  Variable Time Delay30/1 -> Add/32
  Gain21/1 -> Variable Time Delay21/2
  Variable Time Delay28/1 -> Add/30
  Variable Time Delay27/1 -> Add/29
  Gain17/1 -> Variable Time Delay16/2
  Signal_in1/1 -> Gain59/1, Gain14/1, Gain16/1, Gain17/1, Gain18/1, Gain19/1, Gain30/1, Gain21/1, Gain22/1, Gain23/1, Gain24/1, Gain25/1, Gain29/1, Gain40/1, Gain31/1, Gain32/1, Gain33/1, Gain34/1, Gain35/1, Gain36/1, Gain37/1, Gain38/1, Gain50/1, Gain41/1, Gain42/1, Gain43/1, Gain44/1, Gain45/1, Gain46/1, Gain47/1, Gain48/1, Gain2/1, Gain57/1, Gain58/1, Gain56/1, Gain55/1, Gain54/1, Gain53/1, Gain52/1, Gain51/1, Gain3/1, Gain49/1, Gain39/1, Gain28/1, Gain27/1, Gain26/1, Gain20/1, Gain15/1, Gain13/1, Gain12/1, Gain60/1, Gain9/1, Gain8/1, Gain7/1, Gain6/1, Gain5/1, Gain4/1, Gain1/1, Gain/1, Variable Time Delay/2
  Variable Time Delay11/1 -> Add/13
  Gain25/1 -> Variable Time Delay25/2
  Gain59/1 -> Variable Time Delay50/2
  Variable Time Delay52/1 -> Add/53
  Gain41/1 -> Variable Time Delay41/2
  Gain22/1 -> Variable Time Delay22/2
  Variable Time Delay16/1 -> Add/18
  Gain54/1 -> Variable Time Delay56/2
  Gain58/1 -> Variable Time Delay60/2
  Variable Time Delay23/1 -> Add/25
  Gain4/1 -> Variable Time Delay4/2
  Variable Time Delay/1 -> Scope3/1, Add/2
  Variable Time Delay51/1 -> Add/52
  Gain38/1 -> Variable Time Delay38/2
  Gain23/1 -> Variable Time Delay23/2
  Variable Time Delay42/1 -> Add/44
  Variable Time Delay9/1 -> Add/10
  Variable Time Delay59/1 -> Add/60
  Gain55/1 -> Variable Time Delay57/2
  Variable Time Delay38/1 -> Add/40
  [sig] -> Variable Time Delay4/1, Variable Time Delay5/1, Variable Time Delay7/1, Variable Time Delay9/1, Variable Time Delay60/1, Variable Time Delay59/1, Variable Time Delay58/1, Variable Time Delay57/1, Variable Time Delay56/1, Variable Time Delay55/1, Variable Time Delay54/1, Variable Time Delay53/1, Variable Time Delay52/1, Variable Time Delay51/1, Variable Time Delay49/1, Variable Time Delay48/1, Variable Time Delay47/1, Variable Time Delay46/1, Variable Time Delay45/1, Variable Time Delay44/1, Variable Time Delay43/1, Variable Time Delay42/1, Variable Time Delay41/1, Variable Time Delay40/1, Variable Time Delay39/1, Variable Time Delay38/1, Variable Time Delay37/1, Variable Time Delay36/1, Variable Time Delay35/1, Variable Time Delay34/1, Variable Time Delay33/1, Variable Time Delay32/1, Variable Time Delay31/1, Variable Time Delay30/1, Variable Time Delay29/1, Variable Time Delay28/1, Variable Time Delay27/1, Variable Time Delay26/1, Variable Time Delay25/1, Variable Time Delay24/1, Variable Time Delay23/1, Variable Time Delay22/1, Variable Time Delay21/1, Variable Time Delay20/1, Variable Time Delay19/1, Variable Time Delay18/1, Variable Time Delay17/1, Variable Time Delay16/1, Variable Time Delay15/1, Variable Time Delay14/1, Variable Time Delay13/1, Variable Time Delay12/1, Variable Time Delay11/1, Variable Time Delay2/1, Variable Time Delay50/1, Variable Time Delay8/1, Variable Time Delay6/1, Variable Time Delay3/1, Variable Time Delay1/1, Variable Time Delay/1, Scope4/1, Scope24/1
  Gain49/1 -> Variable Time Delay49/2
  Variable Time Delay60/1 -> Add/61
  Gain35/1 -> Variable Time Delay35/2
  Variable Time Delay21/1 -> Add/23
  Variable Time Delay49/1 -> Add/51
  Variable Time Delay40/1 -> Add/42
  Gain43/1 -> Variable Time Delay43/2
  Variable Time Delay26/1 -> Add/28
  Gain30/1 -> Variable Time Delay20/2
  Gain39/1 -> Variable Time Delay39/2
  Variable Time Delay41/1 -> Add/43
  Gain50/1 -> Variable Time Delay40/2
  Gain29/1 -> Variable Time Delay29/2
  Gain28/1 -> Variable Time Delay28/2
  Variable Time Delay25/1 -> Add/27
  Gain51/1 -> Variable Time Delay53/2
  Gain14/1 -> Variable Time Delay13/2
  Gain47/1 -> Variable Time Delay47/2
  Gain18/1 -> Variable Time Delay17/2
  Variable Time Delay43/1 -> Add/45
  Constant1/1 -> Divide4/1
  Clock1/1 -> Divide4/2
  Gain10/1 -> Divide5/2
  Step1/1 -> Scope7/1, Divide5/1
  Divide3/1 -> Scope1/1, Gain10/1
  Variable Time Delay81/1 -> Add/1
  Divide5/1 -> Scope5/1, Variable Time Delay81/1, [sig]
  Constant2/1 -> Variable Time Delay81/2
  Divide4/1 -> Math Function1/1
  Sine Wave2/1 -> Divide3/1
  Math Function1/1 -> Scope6/1, Divide3/2

== system ULInjurySubject_Biphasic_1Hz_08102023/excitatory Neuron 1 ==
  Iext : Inport
  "I " : Inport  Port=2
  VPreE7 : Inport  Port=3
  Add : Sum  Inputs=+---+-
  Add1 : Sum  Inputs=+-
  Constant2 : Constant  Value=ENaEx
  Divide : Product  Inputs=**
  Gain : Gain  Gain=1/Cn
  Integrator : Integrator  InitialCondition=-65  AbsoluteTolerance=1e-6
  Ks : Subsystem
  Lk : Subsystem
  Naf : Subsystem
  Nap1 : Subsystem
  Scope{1..3,5} (4 alike) : Scope
  Subsystem : Subsystem
  Transfer Fcn1 : TransferFcn  Denominator=[TawIExt 1]
  Vm : Outport  VectorParamsAs1DForOutWhenUnconnected=off
  wires:
  Divide/1 -> Add/1
  Ks/1(IKs) -> Add/3
  Naf/1("INaf ") -> Add/2
  Add/1 -> Scope3/1, Gain/1
  Transfer Fcn1/1 -> Divide/2, Scope1/1
  Gain/1 -> Integrator/1
  Subsystem/1(ku) -> Transfer Fcn1/1
  Iext/1 -> Subsystem/1(Iext)
  "I "/1 -> Add/5
  Add1/1 -> Divide/1
  Constant2/1 -> Add1/1
  Integrator/1 -> Naf/1(Vm), Add1/2, Ks/1(Vm), Lk/1(Vm), Nap1/1(V), Vm/1
  Nap1/1("ISynE ") -> Add/6, Scope2/1
  VPreE7/1 -> Nap1/2(Pre)
  Lk/1(ILk) -> Scope5/1, Add/4

== system ULInjurySubject_Biphasic_1Hz_08102023/excitatory Neuron 1-1 ==
  Iext : Inport
  VPreE1 : Inport  Port=2
  Add : Sum  Inputs=+----
  Add1 : Sum  Inputs=+-
  Constant2 : Constant  Value=ENaEx
  Divide : Product  Inputs=**
  Gain : Gain  Gain=1/Cn
  Integrator : Integrator  InitialCondition=V0
  Ks : Subsystem
  Lk : Subsystem
  Naf : Subsystem
  Nap1 : Subsystem
  Scope{1..3,5} (4 alike) : Scope
  Subsystem : Subsystem
  Transfer Fcn1 : TransferFcn  Denominator="[TawIExtE  1]"
  Vm : Outport  VectorParamsAs1DForOutWhenUnconnected=off
  wires:
  Divide/1 -> Add/1
  Ks/1(IKs) -> Add/3
  Naf/1("INaf ") -> Add/2
  Add/1 -> Scope3/1, Gain/1
  Transfer Fcn1/1 -> Divide/2, Scope1/1
  Gain/1 -> Integrator/1
  Subsystem/1(ku) -> Transfer Fcn1/1
  Iext/1 -> Subsystem/1(Iext)
  Add1/1 -> Divide/1
  Constant2/1 -> Add1/1
  Integrator/1 -> Lk/1(Vm), Ks/1(Vm), Naf/1(Vm), Add1/2, Nap1/1(V), Vm/1
  VPreE1/1 -> Nap1/2(Pre)
  Lk/1(ILk) -> Add/4, Scope5/1
  Nap1/1("ISynE ") -> Add/5

== system ULInjurySubject_Biphasic_1Hz_08102023/excitatory Neuron 2 ==
  Iext : Inport
  "I " : Inport  Port=2
  "VPre1I " : Inport  Port=3
  VPre6E : Inport  Port=4
  VPre1I : Inport  Port=5
  VPre8E : Inport  Port=6
  Add : Sum  Inputs=+---++----
  Add1 : Sum  Inputs=+-
  Constant2 : Constant  Value=ENaEx
  Divide : Product  Inputs=**
  Gain : Gain  Gain=1/Cn
  Integrator : Integrator  InitialCondition=V0
  Ks : Subsystem
  Lk : Subsystem
  Naf : Subsystem
  Nap1 : Subsystem
  Nap2 : Subsystem
  Nap3 : Subsystem
  Nap4 : Subsystem
  Scope{1..3,5} (4 alike) : Scope
  Subsystem : Subsystem
  Transfer Fcn1 : TransferFcn  Denominator=[TawIExtE 1]
  Vm : Outport  VectorParamsAs1DForOutWhenUnconnected=off
  wires:
  Divide/1 -> Add/1
  Ks/1(IKs) -> Add/3
  Naf/1("INaf ") -> Add/2
  Add/1 -> Scope3/1, Gain/1
  Lk/1(ILk) -> Add/4, Scope5/1
  Transfer Fcn1/1 -> Divide/2, Scope1/1
  Gain/1 -> Integrator/1
  Subsystem/1(ku) -> Transfer Fcn1/1
  Iext/1 -> Subsystem/1(Iext)
  "I "/1 -> Add/5
  Add1/1 -> Divide/1
  Constant2/1 -> Add1/1
  Integrator/1 -> Nap4/1(V), Nap1/1(V), Add1/2, Naf/1(Vm), Ks/1(Vm), Lk/1(Vm), Nap2/1(V), Nap3/1(V), Vm/1
  Nap2/1("ISynI ") -> Add/8
  Nap1/1("ISynE ") -> Scope2/1, Add/7
  VPre8E/1 -> Nap4/2(Pre2)
  VPre1I/1 -> Nap3/2(Pre)
  Nap4/1("ISynE ") -> Add/10
  VPre6E/1 -> Nap1/2(Pre2)
  "VPre1I "/1 -> Nap2/2(Pre)

== system ULInjurySubject_Biphasic_1Hz_08102023/excitatory Neuron 3 ==
  Iext : Inport
  "I " : Inport  Port=2
  "VPreI " : Inport  Port=3
  VPre8E : Inport  Port=4
  Add : Sum  Inputs=+---++--
  Add1 : Sum  Inputs=+-
  Constant2 : Constant  Value=ENaEx
  Divide : Product  Inputs=**
  Gain : Gain  Gain=1/Cn
  Integrator : Integrator  InitialCondition=V0
  Ks : Subsystem
  Lk : Subsystem
  Naf : Subsystem
  Nap4 : Subsystem
  Nap5 : Subsystem
  Scope{1..8} (8 alike) : Scope
  Subsystem : Subsystem
  Transfer Fcn1 : TransferFcn  Denominator=[TawIExt 1]
  Vm : Outport  VectorParamsAs1DForOutWhenUnconnected=off
  wires:
  Divide/1 -> Add/1
  Ks/1(IKs) -> Scope4/1, Add/3
  Naf/1("INaf ") -> Scope6/1, Add/2
  Add/1 -> Scope3/1, Gain/1
  Lk/1(ILk) -> Add/4, Scope5/1
  Transfer Fcn1/1 -> Divide/2, Scope1/1
  Gain/1 -> Integrator/1
  Subsystem/1(ku) -> Transfer Fcn1/1
  Iext/1 -> Subsystem/1(Iext)
  "I "/1 -> Add/5
  Add1/1 -> Divide/1
  Constant2/1 -> Add1/1
  VPre8E/1 -> Nap5/2(Pre)
  Integrator/1 -> Scope2/1, Nap4/1(V), Lk/1(Vm), Ks/1(Vm), Naf/1(Vm), Add1/2, Nap5/1(V), Vm/1
  "VPreI "/1 -> Nap4/2(Pre)
  Nap4/1("ISynI ") -> Scope8/1, Add/7
  Nap5/1("ISynE ") -> Scope7/1, Add/8

== system ULInjurySubject_Biphasic_1Hz_08102023/excitatory Neuron 4 ==
  "I " : Inport
  "VPre1E " : Inport  Port=2
  VPre3E : Inport  Port=3
  Iext : Inport  Port=4
  Add : Sum  Inputs=+---++----
  Add1 : Sum  Inputs=+-
  Constant2 : Constant  Value=ENaEx
  Divide : Product  Inputs=**
  Gain : Gain  Gain=1/Cn
  Integrator : Integrator  InitialCondition=-65
  Ks : Subsystem
  Lk : Subsystem
  Naf : Subsystem
  Nap1 : Subsystem
  Nap3 : Subsystem
  Scope{1..5} (5 alike) : Scope
  Subsystem : Subsystem
  Transfer Fcn1 : TransferFcn  Denominator=[TawIExt 1]
  Vm : Outport  VectorParamsAs1DForOutWhenUnconnected=off
  wires:
  Divide/1 -> Add/1
  Ks/1(IKs) -> Add/3
  Naf/1("INaf ") -> Add/2
  Add/1 -> Scope3/1, Gain/1
  Lk/1(ILk) -> Add/4, Scope5/1
  Gain/1 -> Integrator/1
  VPre3E/1 -> Nap3/2(Pre)
  Nap1/1("ISynE ") -> Add/7
  Nap3/1("ISynE ") -> Scope4/1, Add/9
  Integrator/1 -> Scope2/1, Nap3/1(V), Naf/1(Vm), Ks/1(Vm), Lk/1(Vm), Nap1/1(V), Vm/1
  "VPre1E "/1 -> Nap1/2(Pre)
  Subsystem/1(ku) -> Transfer Fcn1/1
  "I "/1 -> Add/5, Add1/2
  Add1/1 -> Divide/1
  Constant2/1 -> Add1/1
  Transfer Fcn1/1 -> Divide/2, Scope1/1
  Iext/1 -> Subsystem/1(Iext)

== system ULInjurySubject_Biphasic_1Hz_08102023/excitatory Neuron 6_1 ==
  Iext : Inport
  VPre6E : Inport  Port=2
  Add : Sum  Inputs=+----
  Add1 : Sum  Inputs=+-
  Constant2 : Constant  Value=ENaEx
  Divide : Product  Inputs=**
  Gain : Gain  Gain=1/Cn
  Integrator : Integrator  InitialCondition=-65
  Ks : Subsystem
  Lk : Subsystem
  Naf : Subsystem
  Nap1 : Subsystem
  Scope{1..7} (7 alike) : Scope
  Subsystem : Subsystem
  Transfer Fcn1 : TransferFcn  Denominator="[TawIExtE  1]"
  Vm : Outport  VectorParamsAs1DForOutWhenUnconnected=off
  wires:
  Divide/1 -> Add/1
  Ks/1(IKs) -> Scope6/1, Add/3
  Naf/1("INaf ") -> Scope7/1, Add/2
  Add/1 -> Scope3/1, Gain/1
  Lk/1(ILk) -> Scope5/1, Add/4
  Transfer Fcn1/1 -> Divide/2, Scope1/1
  Gain/1 -> Integrator/1
  Subsystem/1(ku) -> Scope4/1, Transfer Fcn1/1
  Iext/1 -> Subsystem/1(Iext)
  Add1/1 -> Divide/1
  Constant2/1 -> Add1/1
  Integrator/1 -> Vm/1, Nap1/1(V), Add1/2, Naf/1(Vm), Ks/1(Vm), Lk/1(Vm), Scope2/1
  VPre6E/1 -> Nap1/2(Pre)
  Nap1/1("ISynE ") -> Add/5

== system ULInjurySubject_Biphasic_1Hz_08102023/Inhibitory Neuron 10/Ks ==
  Vm : Inport
  Add : Sum  Inputs=-+
  Constant : Constant  Value=gKIn
  Constant1 : Constant  Value=EKIn
  Divide : Product  Inputs=*****
  Divide1 : Product  Inputs=**
  "n " : Subsystem
  IKs : Outport  VectorParamsAs1DForOutWhenUnconnected=off
  wires:
  Constant1/1 -> Add/1
  Add/1 -> Divide1/2
  Divide1/1 -> IKs/1
  Divide/1 -> Divide1/1
  [Vm] -> "n "/1(Vm)
  Vm/1 -> Add/2, [Vm]
  Constant/1 -> Divide/5
  "n "/1(n) -> Divide/3, Divide/4, Divide/2, Divide/1

== system ULInjurySubject_Biphasic_1Hz_08102023/Inhibitory Neuron 10/Lk ==
  Vm : Inport
  Add : Sum  Inputs=-+
  Constant : Constant  Value=gLIn
  Constant1 : Constant  Value=ELIn
  Divide1 : Product  Inputs=**
  ILk : Outport  VectorParamsAs1DForOutWhenUnconnected=off
  wires:
  Constant1/1 -> Add/1
  Add/1 -> Divide1/2
  Divide1/1 -> ILk/1
  Vm/1 -> Add/2, [Vm]
  Constant/1 -> Divide1/1

== system ULInjurySubject_Biphasic_1Hz_08102023/Inhibitory Neuron 10/Naf ==
  Vm : Inport
  Add : Sum  Inputs=-+
  Constant : Constant  Value=gNaIn
  Constant1 : Constant  Value=ENaIn
  Divide : Product  Inputs=*****
  Divide1 : Product  Inputs=**
  h : Subsystem
  "m " : Subsystem
  "INaf " : Outport  VectorParamsAs1DForOutWhenUnconnected=off
  wires:
  Constant1/1 -> Add/1
  Constant/1 -> Divide/5
  Add/1 -> Divide1/2
  [Vm] -> h/1(Vi)
  Divide1/1 -> "INaf "/1
  "m "/1(mNaf) -> Divide/3, Divide/2, Divide/1
  h/1(hNaf) -> Divide/4
  Divide/1 -> Divide1/1
  [Vm] -> "m "/1(Vm)
  Vm/1 -> Add/2, [Vm]

== system ULInjurySubject_Biphasic_1Hz_08102023/Inhibitory Neuron 10/Nap2 ==
  V : Inport
  Pre : Inport  Port=2
  Add : Sum  Inputs=-+
  Add1 : Sum  Inputs=+-
  Constant : Constant  Value=gSynE6
  Constant1 : Constant  Value=ESynE610
  Constant3 : Constant  Value=w10
  Constant4 : Constant  Value=-65
  Divide : Product  Inputs=**
  Divide1 : Product  Inputs=***
  Saturation : Saturate  UpperLimit=inf  LowerLimit=0
  Saturation1 : Saturate  UpperLimit=inf  LowerLimit=0
  Scope : Scope
  Scope1 : Scope
  Transfer Fcn : TransferFcn  Denominator=[TawSynE10 1]
  "ISynE " : Outport  VectorParamsAs1DForOutWhenUnconnected=off
  wires:
  Constant1/1 -> Add/1
  Divide1/1 -> "ISynE "/1
  Constant/1 -> Divide1/1
  V/1 -> Add/2
  Constant3/1 -> Saturation/1
  Saturation/1 -> Divide/1
  Divide/1 -> Divide1/3
  Transfer Fcn/1 -> Scope/1, Divide/2
  Pre/1 -> Add1/1
  Add1/1 -> Saturation1/1
  Constant4/1 -> Add1/2
  Add/1 -> Scope1/1, Divide1/2
  Saturation1/1 -> Transfer Fcn/1

== system ULInjurySubject_Biphasic_1Hz_08102023/Inhibitory Neuron 10/Subsystem ==
  Iext : Inport
  Constant1 : Constant  Value=1/30
  Divide2 : Product  Inputs=**
  ku : Outport  VectorParamsAs1DForOutWhenUnconnected=off
  wires:
  Divide2/1 -> ku/1
  Constant1/1 -> Divide2/2
  Iext/1 -> Divide2/1
